simulink model "LinearEQTNSimulink2"  (Simulink 7.0)
settings: Solver=ode45  StartTime=0.0  StopTime=10.0  RelTol=1e-3
settings Model: Creator=Ben Favour  LastModifiedBy=Ben Favour

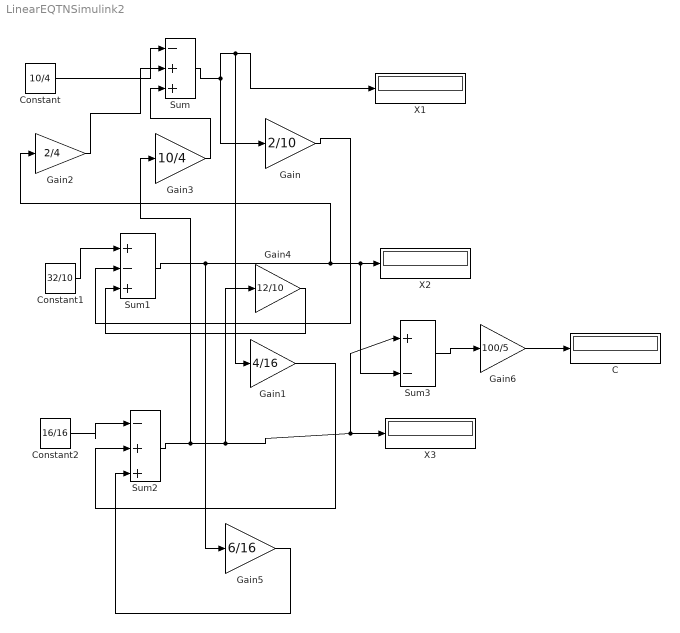
== system LinearEQTNSimulink2 ==
  C : Display
  Constant : Constant  Value=10/4  OutDataType=sfix(16)  OutScaling=2^0
  Constant1 : Constant  Value=32/10  OutDataType=sfix(16)  OutScaling=2^0
  Constant2 : Constant  Value=16/16  OutDataType=sfix(16)  OutScaling=2^0
  Gain : Gain  Gain=2/10  ParameterDataType=sfix(16)  ParameterScaling=2^0  OutDataType=sfix(16)  OutScaling=2^0
  Gain1 : Gain  Gain=4/16  ParameterDataType=sfix(16)  ParameterScaling=2^0  OutDataType=sfix(16)  OutScaling=2^0
  Gain2 : Gain  Gain=2/4  ParameterDataType=sfix(16)  ParameterScaling=2^0  OutDataType=sfix(16)  OutScaling=2^0
  Gain3 : Gain  Gain=10/4  ParameterDataType=sfix(16)  ParameterScaling=2^0  OutDataType=sfix(16)  OutScaling=2^0
  Gain4 : Gain  Gain=12/10  ParameterDataType=sfix(16)  ParameterScaling=2^0  OutDataType=sfix(16)  OutScaling=2^0
  Gain5 : Gain  Gain=6/16  ParameterDataType=sfix(16)  ParameterScaling=2^0  OutDataType=sfix(16)  OutScaling=2^0
  Gain6 : Gain  Gain=100/5  ParameterDataType=sfix(16)  ParameterScaling=2^0  OutDataType=sfix(16)  OutScaling=2^0
  Sum : Sum  Inputs=-++  OutDataType=sfix(16)  OutScaling=2^0
  Sum1 : Sum  Inputs=|+-+  OutDataType=sfix(16)  OutScaling=2^0
  Sum2 : Sum  Inputs=|-++  OutDataType=sfix(16)  OutScaling=2^0
  Sum3 : Sum  Inputs=|+-  OutDataType=sfix(16)  OutScaling=2^0
  X1 : Display
  X2 : Display
  X3 : Display
  wires:
  Constant/1 -> Sum/1
  Sum/1 -> Gain/1, X1/1, Gain1/1
  Constant1/1 -> Sum1/1
  Sum1/1 -> Gain2/1, X2/1, Sum3/2, Gain5/1
  Gain2/1 -> Sum/2
  Gain/1 -> Sum1/2
  Constant2/1 -> Sum2/1
  Sum2/1 -> Gain3/1, Gain4/1, X3/1, Sum3/1
  Gain1/1 -> Sum2/2
  Gain3/1 -> Sum/3
  Gain4/1 -> Sum1/3
  Gain5/1 -> Sum2/3
  Sum3/1 -> Gain6/1
  Gain6/1 -> C/1
